simulink model "car_following_model"  (R2017a)
settings: Solver=FixedStepAuto  StartTime=0.0  StopTime=70  FixedStep=.001  RelTol=1e-3
model workspace (MAT data in the model file):
  t_0 = 0
values from neighbouring files (symbols this model uses):
  a = a_list(a_i)    [critical_tau_epsilon.m]    (also in platooning_model_implementation.m = 1.4; run_simulink.m = 1)
  a_max = 1    [critical_tau_epsilon.m]    (also in platooning_model_implementation.m; run_simulink.m)
  a_min = -0.5    [critical_tau_epsilon.m]    (also in platooning_model_implementation.m; run_simulink.m)
  b = 2.0    (= 2)    [critical_tau_epsilon.m]    (also in platooning_model_implementation.m; run_simulink.m)
  delta = 4    [critical_tau_epsilon.m]    (also in platooning_model_implementation.m; run_simulink.m)
  l_avg = 4.8    [critical_tau_epsilon.m]    (also in platooning_model_implementation.m; run_simulink.m)
  N = 1000    [critical_tau_epsilon.m]    (also in platooning_model_implementation.m; run_simulink.m)
  s_0 = 2.0    (= 2)    [critical_tau_epsilon.m]    (also in platooning_model_implementation.m; run_simulink.m)
  T = 1.5    [critical_tau_epsilon.m]    (also in platooning_model_implementation.m; run_simulink.m)
  v_0 = 120    [critical_tau_epsilon.m]    (also in platooning_model_implementation.m; run_simulink.m)
undefined symbols (not defined in the file or in its folder): canChannel
libraries: canlib x9, canmsglib x7, simulink x1, dspstat3 x1, dspindex x1
settings Model: Creator=s132652  LastModifiedBy=s132652

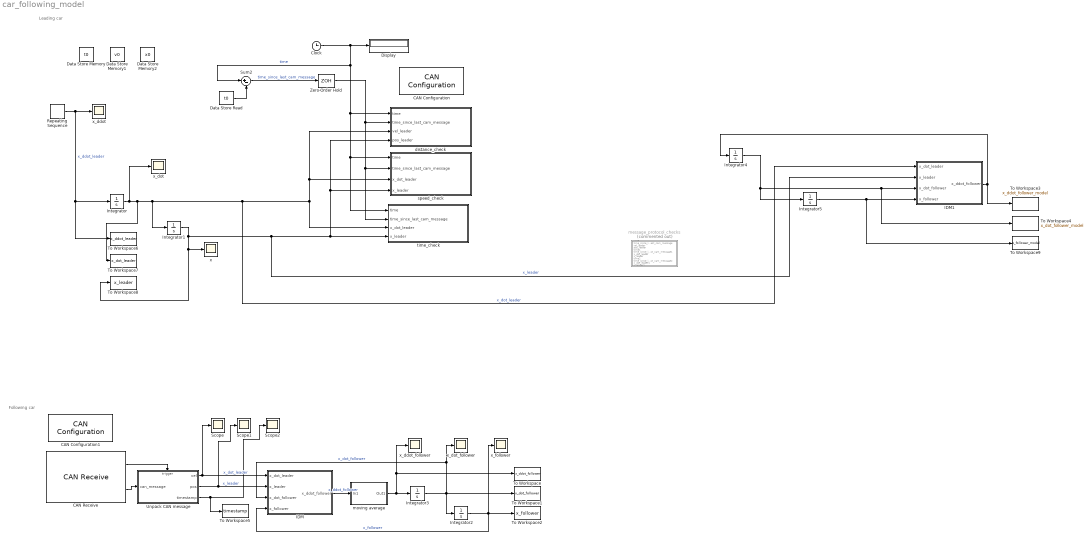
== system car_following_model ==
  note: Leading car
  note: Following car
  CAN Configuration : canlib/CAN Configuration  BlockHandle=5.0001  DeviceMenu=MathWorks Virtual 1 (Channel 1)  Device=MathWorks Virtual 1 (Channel 1)  ObjConstructor=canChannel('MathWorks','Virtual 1',1)  BusSpeed=500000  EnableBitParameters=off  SJW=0  TSEG1=0  TSEG2=0  NSamples=0  AckMode=Normal
      settings: SourceProductName=Vehicle Network Toolbox  SourceProductBaseCode=VN
  CAN Configuration1 : canlib/CAN Configuration  BlockHandle=6.0001  DeviceMenu=MathWorks Virtual 1 (Channel 2)  Device=MathWorks Virtual 1 (Channel 2)  ObjConstructor=canChannel('MathWorks','Virtual 1',2)  BusSpeed=500000  EnableBitParameters=off  SJW=0  TSEG1=0  TSEG2=0  NSamples=0  AckMode=Normal
      settings: SourceProductName=Vehicle Network Toolbox  SourceProductBaseCode=VN
  CAN Receive : canlib/CAN Receive  BlockHandle=7.0001  DeviceMenu=MathWorks Virtual 1 (Channel 2)  Device=MathWorks Virtual 1 (Channel 2)  ObjConstructor=canChannel('MathWorks','Virtual 1',2)  EnableStandardIDsFilter=off  StandardIDs=0  EnableExtendedIDsFilter=off  ExtendedIDs=0  SampleTime=0.01  MsgsPerTimestep=all  StdIDsCombo=Allow all  ExtIDsCombo=Allow all  InternalFilterUpdateStatus=on
      settings: SourceProductName=Vehicle Network Toolbox  SourceProductBaseCode=VN
  Clock : Clock
  Data Store Memory : DataStoreMemory  DataStoreName=t0  ReadBeforeWriteMsg=warning  WriteAfterWriteMsg=warning  WriteAfterReadMsg=warning  ShowAdditionalParam=off
  Data Store Memory1 : DataStoreMemory  DataStoreName=v0  ReadBeforeWriteMsg=warning  WriteAfterWriteMsg=warning  WriteAfterReadMsg=warning  InitialValue=10  ShowAdditionalParam=off
  Data Store Memory2 : DataStoreMemory  DataStoreName=x0  ReadBeforeWriteMsg=warning  WriteAfterWriteMsg=warning  WriteAfterReadMsg=warning  InitialValue=100  ShowAdditionalParam=off
  Data Store Read : DataStoreRead  DataStoreName=t0
  Display : Display
  IDM : Subsystem
  IDM1 : Subsystem
  Integrator : Integrator  InitialCondition=10
  Integrator1 : Integrator  InitialCondition=100
  Integrator2 : Integrator  InitialCondition=76
  Integrator3 : Integrator  InitialCondition=10
  Integrator4 : Integrator  InitialCondition=10
  Integrator5 : Integrator  InitialCondition=78.2
  Repeating Sequence : simulink/Sources/Repeating Sequence  rep_seq_t=[0 5 10 15 20 25 30 35 40 45 50 55 60 65 70]  rep_seq_y=[0 0 0 0 0 a_max a_max 0 0 0 a_min a_min 0 0 0]
  Scope : Scope
  Scope1 : Scope
  Scope2 : Scope
  Sum2 : Sum  Inputs=|+-
  To Workspace : ToWorkspace  VariableName=x_ddot_follower  SaveFormat=Timeseries  SampleTime=-1
  To Workspace1 : ToWorkspace  VariableName=x_dot_follower  SaveFormat=Timeseries  SampleTime=-1
  To Workspace2 : ToWorkspace  VariableName=x_follower  SaveFormat=Timeseries  SampleTime=-1
  To Workspace3 : ToWorkspace  VariableName=x_ddot_follower_model  SaveFormat=Timeseries  SampleTime=-1
  To Workspace4 : ToWorkspace  VariableName=x_dot_follower_model  SaveFormat=Timeseries  SampleTime=-1
  To Workspace5 : ToWorkspace  VariableName=timestamp  SaveFormat=Timeseries  SampleTime=-1
  To Workspace6 : ToWorkspace  VariableName=x_ddot_leader  SaveFormat=Timeseries  SampleTime=-1
  To Workspace7 : ToWorkspace  VariableName=x_dot_leader  SaveFormat=Timeseries  SampleTime=-1
  To Workspace8 : ToWorkspace  VariableName=x_leader  SaveFormat=Timeseries  SampleTime=-1
  To Workspace9 : ToWorkspace  VariableName=x_follower_model  SaveFormat=Timeseries  SampleTime=-1
  Unpack CAN message : Subsystem  TreatAsAtomicUnit=on
  Zero-Order Hold : ZeroOrderHold  SampleTime=0.001
  distance_check : Subsystem
  message_protocol_checks : Subsystem  Commented=on
  moving average : Subsystem
  speed_check : Subsystem
  time_check : Subsystem
  x : Scope
  x_ddot : Scope
  x_ddot_follower : Scope
  x_dot : Scope
  x_dot_follower : Scope
  x_follower : Scope
  wires:
  Repeating Sequence/1 -> To Workspace6/1, Integrator/1, x_ddot/1  "x_ddot_leader"
  Integrator/1 -> x_dot/1, To Workspace7/1, Integrator1/1, IDM1/1(x_dot_leader), distance_check/3(vel_leader), speed_check/3(x_dot_leader), time_check/3(x_dot_leader)  "x_dot_leader"
  Integrator1/1 -> To Workspace8/1, x/1, IDM1/2(x_leader), distance_check/4(pos_leader), speed_check/4(x_leader), time_check/4(x_leader)  "x_leader"
  Clock/1 -> time_check/1(time), speed_check/1(time), distance_check/1(time), Sum2/1, Display/1  "time"
  Data Store Read/1 -> Sum2/2
  Sum2/1 -> Zero-Order Hold/1  "time_since_last_cam_message"
  Zero-Order Hold/1 -> time_check/2(time_since_last_cam_message), speed_check/2(time_since_last_cam_message), distance_check/2(time_since_last_cam_message)
  CAN Receive/2 -> Unpack CAN message/1(can_message)
  CAN Receive/1 -> Unpack CAN message/Trigger
  Unpack CAN message/1(vel) -> IDM/1(x_dot_leader), Scope/1  "x_dot_leader"
  Unpack CAN message/2(pos) -> IDM/2(x_leader), Scope1/1  "x_leader"
  Unpack CAN message/3(timestamp) -> To Workspace5/1, Scope2/1
  IDM/1(x_ddot_follower) -> moving average/1(In1)  "x_ddot_follower"
  moving average/1(Out1) -> To Workspace/1, x_ddot_follower/1, Integrator3/1
  Integrator3/1 -> IDM/3(x_dot_follower), x_dot_follower/1, To Workspace1/1, Integrator2/1  "x_dot_follower"
  Integrator2/1 -> To Workspace2/1, IDM/4(x_follower), x_follower/1  "x_follower"
  Integrator4/1 -> To Workspace4/1, IDM1/3(x_dot_follower), Integrator5/1
  Integrator5/1 -> To Workspace9/1, IDM1/4(x_follower)
  IDM1/1(x_ddot_follower) -> To Workspace3/1, Integrator4/1

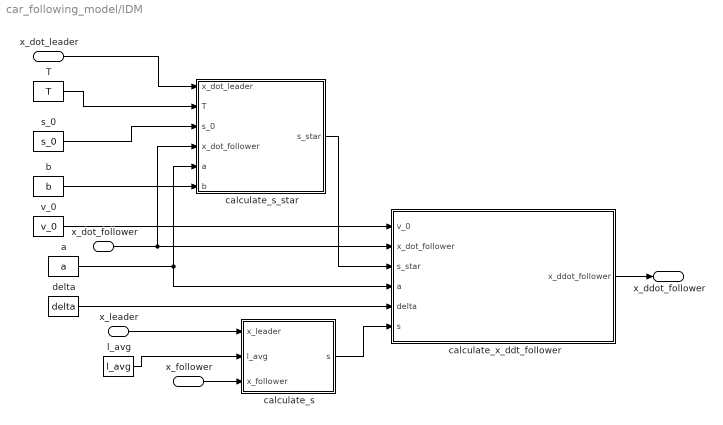
== system car_following_model/IDM ==
  x_dot_leader : Inport
  x_leader : Inport  Port=2
  x_dot_follower : Inport  Port=3
  x_follower : Inport  Port=4
  T : Constant  Value=T
  a : Constant  Value=a
  b : Constant  Value=b
  calculate_s : Subsystem
  calculate_s_star : Subsystem
  calculate_x_ddt_follower : Subsystem
  delta : Constant  Value=delta
  l_avg : Constant  Value=l_avg
  s_0 : Constant  Value=s_0
  v_0 : Constant  Value=v_0
  x_ddot_follower : Outport
  wires:
  v_0/1 -> calculate_x_ddt_follower/1(v_0)
  T/1 -> calculate_s_star/2(T)
  s_0/1 -> calculate_s_star/3(s_0)
  calculate_x_ddt_follower/1(x_ddot_follower) -> x_ddot_follower/1
  b/1 -> calculate_s_star/6(b)
  l_avg/1 -> calculate_s/2(l_avg)
  calculate_s/1(s) -> calculate_x_ddt_follower/6(s)
  delta/1 -> calculate_x_ddt_follower/5(delta)
  calculate_s_star/1(s_star) -> calculate_x_ddt_follower/3(s_star)
  x_follower/1 -> calculate_s/3(x_follower)
  x_dot_leader/1 -> calculate_s_star/1(x_dot_leader)
  x_leader/1 -> calculate_s/1(x_leader)
  x_dot_follower/1 -> calculate_s_star/4(x_dot_follower), calculate_x_ddt_follower/2(x_dot_follower)
  a/1 -> calculate_x_ddt_follower/4(a), calculate_s_star/5(a)

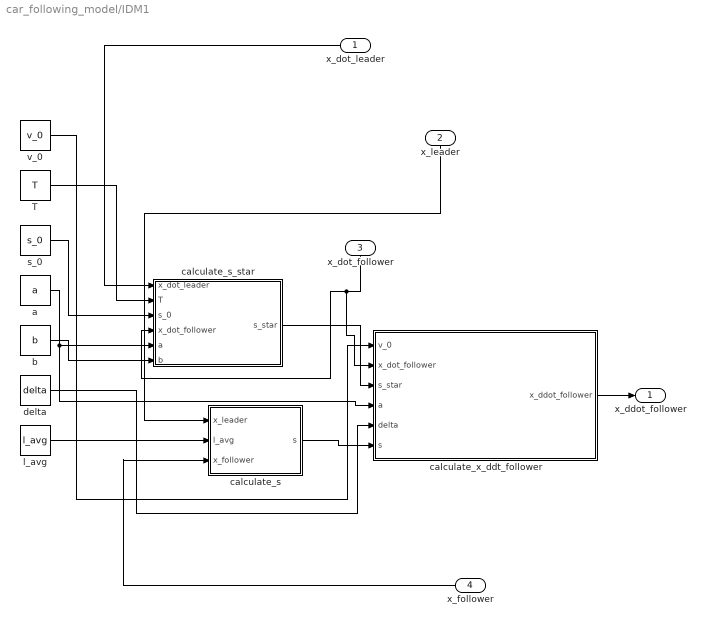
== system car_following_model/IDM1 ==
  x_dot_leader : Inport
  x_leader : Inport  Port=2
  x_dot_follower : Inport  Port=3
  x_follower : Inport  Port=4
  T : Constant  Value=T
  a : Constant  Value=a
  b : Constant  Value=b
  calculate_s : Subsystem
  calculate_s_star : Subsystem
  calculate_x_ddt_follower : Subsystem
  delta : Constant  Value=delta
  l_avg : Constant  Value=l_avg
  "s_0 " : Constant  Value=s_0
  v_0 : Constant  Value=v_0
  x_ddot_follower : Outport
  wires:
  a/1 -> calculate_x_ddt_follower/4(a), calculate_s_star/5(a)
  v_0/1 -> calculate_x_ddt_follower/1(v_0)
  T/1 -> calculate_s_star/2(T)
  "s_0 "/1 -> calculate_s_star/3(s_0)
  calculate_x_ddt_follower/1(x_ddot_follower) -> x_ddot_follower/1
  b/1 -> calculate_s_star/6(b)
  l_avg/1 -> calculate_s/2(l_avg)
  calculate_s/1(s) -> calculate_x_ddt_follower/6(s)
  delta/1 -> calculate_x_ddt_follower/5(delta)
  calculate_s_star/1(s_star) -> calculate_x_ddt_follower/3(s_star)
  x_follower/1 -> calculate_s/3(x_follower)
  x_dot_follower/1 -> calculate_x_ddt_follower/2(x_dot_follower), calculate_s_star/4(x_dot_follower)
  x_dot_leader/1 -> calculate_s_star/1(x_dot_leader)
  x_leader/1 -> calculate_s/1(x_leader)

== system car_following_model/Unpack CAN message ==
  can_message : Inport
  function : TriggerPort  TriggerType=function-call  VariantControl=Variant
  CAN Unpack : canmsglib/CAN Unpack  MsgList=(none)  MsgName=CAN Msg  MsgIDType=Standard (11-bit identifier)  MsgIdentifier=0  MsgLength=8  SignalInfo=position_leader$0$16$1$1$1$0$0.1$0$-Inf$Inf$#velocity_leader$16$16$1$1$1$0$0.0025$0$-Inf$Inf$#timestamp$32$16$1$1$1$0$0.01$0$-Inf$Inf$#  NSignals=3  IDPort=off  TimestampPort=off  ErrorPort=off  RemotePort=off  LengthPort=off  StatusPort=off  StartBits=str2num('[int32(0);int32(16);int32(32)]')  SignalSizes=str2num('[int32(16);int32(16);int32(16)]')  ByteOrders=str2num('[int32(1);int32(1);int32(1)]')  DataTypes=str2num('[int32(1);int32(1);int32(1)]')  MultiplexTypes=str2num('[int32(1);int32(1);int32(1)]')  MultiplexValues=str2num('[double(0);double(0);double(0)]')  Factors=str2num('[double(0.1);double(0.0025);double(0.01)]')  Offsets=str2num('[double(0);double(0);double(0)]')  Minimums=str2num('[double(-Inf);double(-Inf);double(-Inf)]')  Maximums=str2num('[double(Inf);double(Inf);double(Inf)]')  ApplyMinMax=off
      settings: SourceProductName=Simulink Real-Time
  vel : Outport
  pos : Outport  Port=2
  timestamp : Outport  Port=3
  wires:
  can_message/1 -> CAN Unpack/1
  CAN Unpack/2 -> vel/1
  CAN Unpack/1 -> pos/1
  CAN Unpack/3 -> timestamp/1

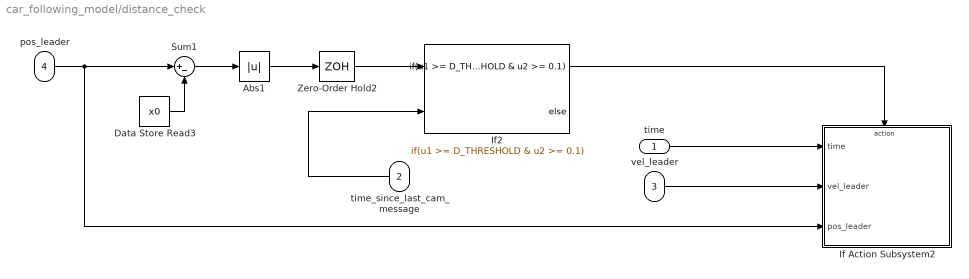
== system car_following_model/distance_check ==
  time : Inport
  time_since_last_cam_message : Inport  Port=2
  vel_leader : Inport  Port=3
  pos_leader : Inport  Port=4
  Abs1 : Abs
  Data Store Read3 : DataStoreRead  DataStoreName=x0
  If Action Subsystem2 : Subsystem  TreatAsAtomicUnit=on
  If2 : If  NumInputs=2  IfExpression=u1 >= D_THRESHOLD & u2 >= 0.1
  Sum1 : Sum  Inputs=|+-
  Zero-Order Hold2 : ZeroOrderHold  SampleTime=0.001
  wires:
  Data Store Read3/1 -> Sum1/2
  Sum1/1 -> Abs1/1
  Abs1/1 -> Zero-Order Hold2/1
  Zero-Order Hold2/1 -> If2/1
  If2/1 -> If Action Subsystem2/Action
  time_since_last_cam_message/1 -> If2/2
  time/1 -> If Action Subsystem2/1(time)
  pos_leader/1 -> If Action Subsystem2/3(pos_leader), Sum1/1
  vel_leader/1 -> If Action Subsystem2/2(vel_leader)

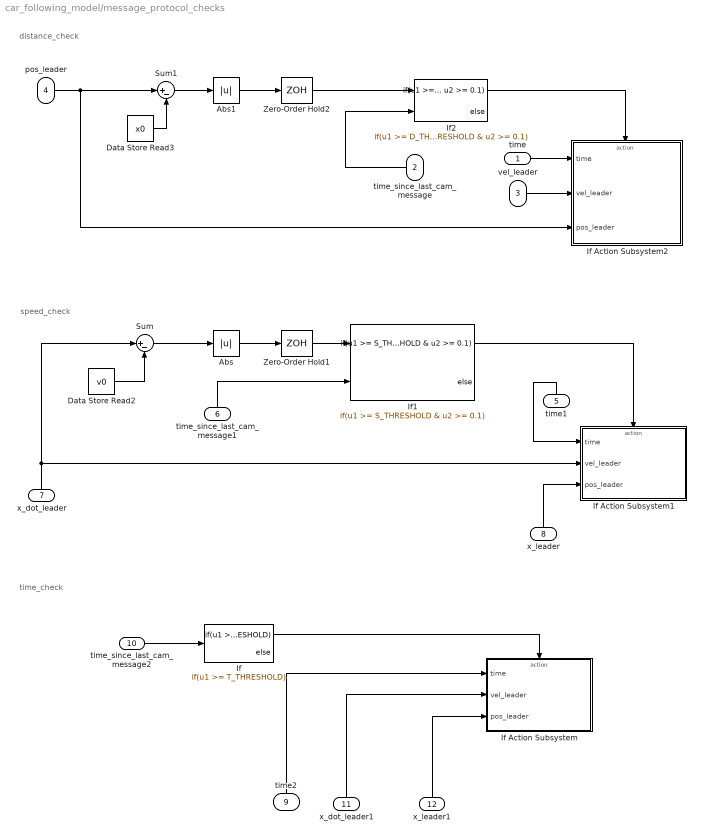
== system car_following_model/message_protocol_checks ==
  note: time_check
  note: speed_check
  note: distance_check
  time : Inport
  time_since_last_cam_message : Inport  Port=2
  vel_leader : Inport  Port=3
  pos_leader : Inport  Port=4
  time1 : Inport  Port=5
  time_since_last_cam_message1 : Inport  Port=6
  x_dot_leader : Inport  Port=7
  x_leader : Inport  Port=8
  time2 : Inport  Port=9
  time_since_last_cam_message2 : Inport  Port=10
  x_dot_leader1 : Inport  Port=11
  x_leader1 : Inport  Port=12
  Abs : Abs
  Abs1 : Abs
  Data Store Read2 : DataStoreRead  DataStoreName=v0
  Data Store Read3 : DataStoreRead  DataStoreName=x0
  If : If  IfExpression=u1 >= T_THRESHOLD
  If Action Subsystem : Subsystem  TreatAsAtomicUnit=on
  If Action Subsystem1 : Subsystem  TreatAsAtomicUnit=on
  If Action Subsystem2 : Subsystem  TreatAsAtomicUnit=on
  If1 : If  NumInputs=2  IfExpression=u1 >= S_THRESHOLD & u2 >= 0.1
  If2 : If  NumInputs=2  IfExpression=u1 >= D_THRESHOLD & u2 >= 0.1
  Sum : Sum  Inputs=|+-
  Sum1 : Sum  Inputs=|+-
  Zero-Order Hold1 : ZeroOrderHold  SampleTime=0.001
  Zero-Order Hold2 : ZeroOrderHold  SampleTime=0.001
  wires:
  time_since_last_cam_message/1 -> If2/2
  If2/1 -> If Action Subsystem2/Action
  Sum1/1 -> Abs1/1
  time/1 -> If Action Subsystem2/1(time)
  Zero-Order Hold2/1 -> If2/1
  Abs1/1 -> Zero-Order Hold2/1
  pos_leader/1 -> If Action Subsystem2/3(pos_leader), Sum1/1
  Data Store Read3/1 -> Sum1/2
  vel_leader/1 -> If Action Subsystem2/2(vel_leader)
  Abs/1 -> Zero-Order Hold1/1
  time1/1 -> If Action Subsystem1/1(time)
  x_dot_leader/1 -> Sum/1, If Action Subsystem1/2(vel_leader)
  Zero-Order Hold1/1 -> If1/1
  Sum/1 -> Abs/1
  Data Store Read2/1 -> Sum/2
  x_leader/1 -> If Action Subsystem1/3(pos_leader)
  time_since_last_cam_message1/1 -> If1/2
  If1/1 -> If Action Subsystem1/Action
  time2/1 -> If Action Subsystem/1(time)
  x_dot_leader1/1 -> If Action Subsystem/2(vel_leader)
  If/1 -> If Action Subsystem/Action
  x_leader1/1 -> If Action Subsystem/3(pos_leader)
  time_since_last_cam_message2/1 -> If/1

== system car_following_model/moving average ==
  note: moving average
  In1 : Inport
  IC : InitialCondition  Value=zeros(N,1)
  Mean : dspstat3/Mean  run=off  reset_popup=None  InputProcessing=Columns as channels (frame based)  directionMode=Each column  dimension=1  roiEnable=off  roiType=Rectangles  roiPortion=Entire ROI  roiOutput=Individual statistics for each ROI  roiFlag=off  outputDataTypeStr=Inherit: Same as accumulator  outputLastDataTypeStr=Inherit: Same as accumulator  outputMin=[]  outputMax=[]  roundingMode=Floor  overflowMode=off
  Memory : Memory
  Mux : Mux  Inputs=2
  Variable Selector : dspindex/Variable Selector  NumInputs=1  rowsOrCols=Rows  IdxMode=Fixed  Elements=1:N-1  ZerOneIdxMode=One-based  errmode=Clip Index  FillMode=on  FillValues=0
  Out1 : Outport
  wires:
  In1/1 -> Mux/1
  Mux/1 -> Mean/1, Memory/1
  Memory/1 -> IC/1
  IC/1 -> Variable Selector/1
  Mean/1 -> Out1/1
  Variable Selector/1 -> Mux/2

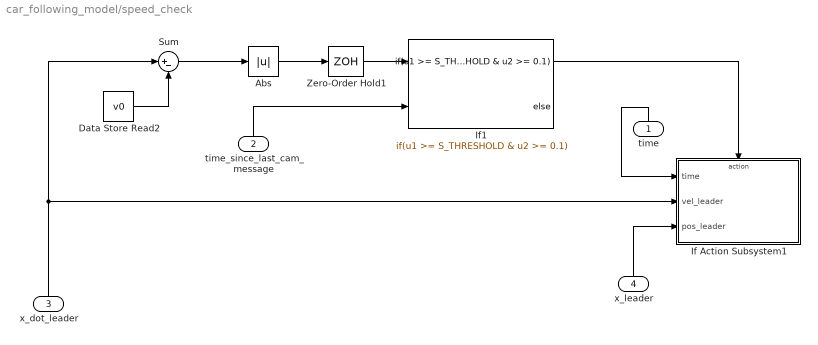
== system car_following_model/speed_check ==
  time : Inport
  time_since_last_cam_message : Inport  Port=2
  x_dot_leader : Inport  Port=3
  x_leader : Inport  Port=4
  Abs : Abs
  Data Store Read2 : DataStoreRead  DataStoreName=v0
  If Action Subsystem1 : Subsystem  TreatAsAtomicUnit=on
  If1 : If  NumInputs=2  IfExpression=u1 >= S_THRESHOLD & u2 >= 0.1
  Sum : Sum  Inputs=|+-
  Zero-Order Hold1 : ZeroOrderHold  SampleTime=0.001
  wires:
  Data Store Read2/1 -> Sum/2
  Sum/1 -> Abs/1
  Abs/1 -> Zero-Order Hold1/1
  If1/1 -> If Action Subsystem1/Action
  Zero-Order Hold1/1 -> If1/1
  time/1 -> If Action Subsystem1/1(time)
  x_dot_leader/1 -> Sum/1, If Action Subsystem1/2(vel_leader)
  x_leader/1 -> If Action Subsystem1/3(pos_leader)
  time_since_last_cam_message/1 -> If1/2

== system car_following_model/time_check ==
  time : Inport
  time_since_last_cam_message : Inport  Port=2
  x_dot_leader : Inport  Port=3
  x_leader : Inport  Port=4
  If : If  IfExpression=u1 >= T_THRESHOLD
  If Action Subsystem : Subsystem  TreatAsAtomicUnit=on
  wires:
  If/1 -> If Action Subsystem/Action
  time_since_last_cam_message/1 -> If/1
  time/1 -> If Action Subsystem/1(time)
  x_dot_leader/1 -> If Action Subsystem/2(vel_leader)
  x_leader/1 -> If Action Subsystem/3(pos_leader)

== system car_following_model/IDM/calculate_s ==
  x_leader : Inport
  l_avg : Inport  Port=2
  x_follower : Inport  Port=3
  Sum3 : Sum  Inputs=|+-
  Sum4 : Sum  Inputs=|+-
  s : Outport
  wires:
  Sum4/1 -> s/1  "s"
  Sum3/1 -> Sum4/1
  l_avg/1 -> Sum4/2
  x_follower/1 -> Sum3/2
  x_leader/1 -> Sum3/1

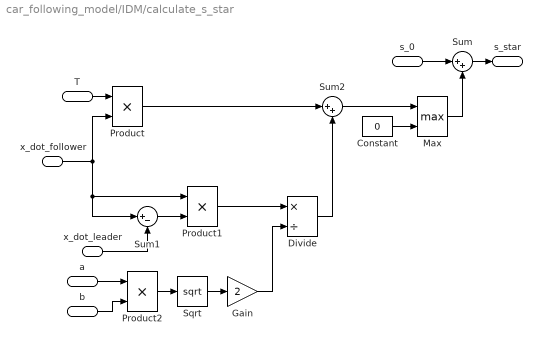
== system car_following_model/IDM/calculate_s_star ==
  x_dot_leader : Inport
  T : Inport  Port=2
  s_0 : Inport  Port=3
  x_dot_follower : Inport  Port=4
  a : Inport  Port=5
  b : Inport  Port=6
  Constant : Constant  Value=0
  Divide : Product  Inputs=*/
  Gain : Gain  Gain=2
  Max : MinMax  Function=max  Inputs=2
  Product : Product
  Product1 : Product
  Product2 : Product
  Sqrt : Sqrt  SaturateOnIntegerOverflow=on
  Sum : Sum  Inputs=|++
  Sum1 : Sum  Inputs=|+-
  Sum2 : Sum  Inputs=|++
  s_star : Outport
  wires:
  Sum1/1 -> Product1/2
  T/1 -> Product/1
  s_0/1 -> Sum/1
  Product1/1 -> Divide/1
  Product/1 -> Sum2/1
  Divide/1 -> Sum2/2
  x_dot_leader/1 -> Sum1/2
  Product2/1 -> Sqrt/1
  Sqrt/1 -> Gain/1
  Gain/1 -> Divide/2
  a/1 -> Product2/1
  b/1 -> Product2/2
  Constant/1 -> Max/2
  Sum2/1 -> Max/1
  Max/1 -> Sum/2
  Sum/1 -> s_star/1
  x_dot_follower/1 -> Product/2, Product1/1, Sum1/1

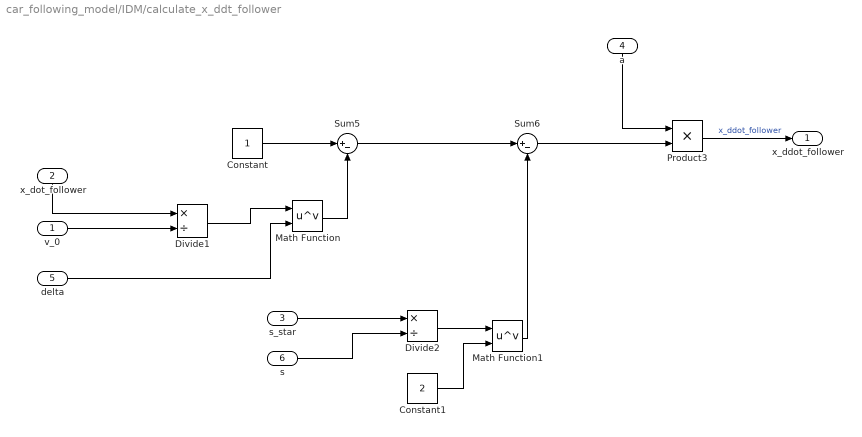
== system car_following_model/IDM/calculate_x_ddt_follower ==
  v_0 : Inport
  x_dot_follower : Inport  Port=2
  s_star : Inport  Port=3
  a : Inport  Port=4
  delta : Inport  Port=5
  s : Inport  Port=6
  Constant : Constant
  Constant1 : Constant  Value=2
  Divide1 : Product  Inputs=*/
  Divide2 : Product  Inputs=*/
  Math Function : Math  Operator=pow  SaturateOnIntegerOverflow=on
  Math Function1 : Math  Operator=pow  SaturateOnIntegerOverflow=on
  Product3 : Product
  Sum5 : Sum  Inputs=|+-
  Sum6 : Sum  Inputs=|+-
  x_ddot_follower : Outport
  wires:
  Product3/1 -> x_ddot_follower/1  "x_ddot_follower"
  v_0/1 -> Divide1/2
  Constant/1 -> Sum5/1
  Math Function/1 -> Sum5/2
  a/1 -> Product3/1
  x_dot_follower/1 -> Divide1/1
  s/1 -> Divide2/2
  s_star/1 -> Divide2/1
  Sum5/1 -> Sum6/1
  Constant1/1 -> Math Function1/2
  Divide1/1 -> Math Function/1
  Math Function1/1 -> Sum6/2
  delta/1 -> Math Function/2
  Divide2/1 -> Math Function1/1
  Sum6/1 -> Product3/2

== system car_following_model/IDM1/calculate_s ==
  x_leader : Inport
  l_avg : Inport  Port=2
  x_follower : Inport  Port=3
  Sum3 : Sum  Inputs=|+-
  Sum4 : Sum  Inputs=|+-
  s : Outport
  wires:
  Sum4/1 -> s/1  "s"
  Sum3/1 -> Sum4/1
  l_avg/1 -> Sum4/2
  x_follower/1 -> Sum3/2
  x_leader/1 -> Sum3/1

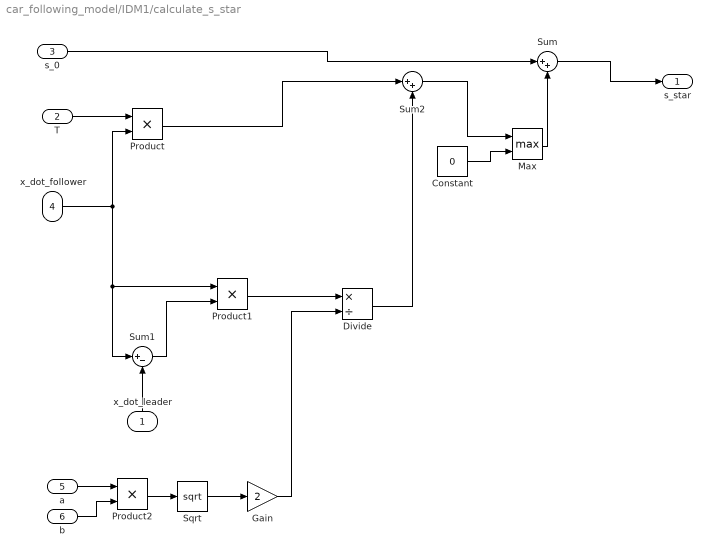
== system car_following_model/IDM1/calculate_s_star ==
  x_dot_leader : Inport
  T : Inport  Port=2
  s_0 : Inport  Port=3
  x_dot_follower : Inport  Port=4
  a : Inport  Port=5
  b : Inport  Port=6
  Constant : Constant  Value=0
  Divide : Product  Inputs=*/
  Gain : Gain  Gain=2
  Max : MinMax  Function=max  Inputs=2
  Product : Product
  Product1 : Product
  Product2 : Product
  Sqrt : Sqrt  SaturateOnIntegerOverflow=on
  Sum : Sum  Inputs=|++
  Sum1 : Sum  Inputs=|+-
  Sum2 : Sum  Inputs=|++
  s_star : Outport
  wires:
  Sum1/1 -> Product1/2
  T/1 -> Product/1
  s_0/1 -> Sum/1
  Product1/1 -> Divide/1
  Product/1 -> Sum2/1
  Divide/1 -> Sum2/2
  x_dot_leader/1 -> Sum1/2
  x_dot_follower/1 -> Product/2, Sum1/1, Product1/1
  Product2/1 -> Sqrt/1
  Sqrt/1 -> Gain/1
  Gain/1 -> Divide/2
  a/1 -> Product2/1
  b/1 -> Product2/2
  Constant/1 -> Max/2
  Sum2/1 -> Max/1
  Max/1 -> Sum/2
  Sum/1 -> s_star/1

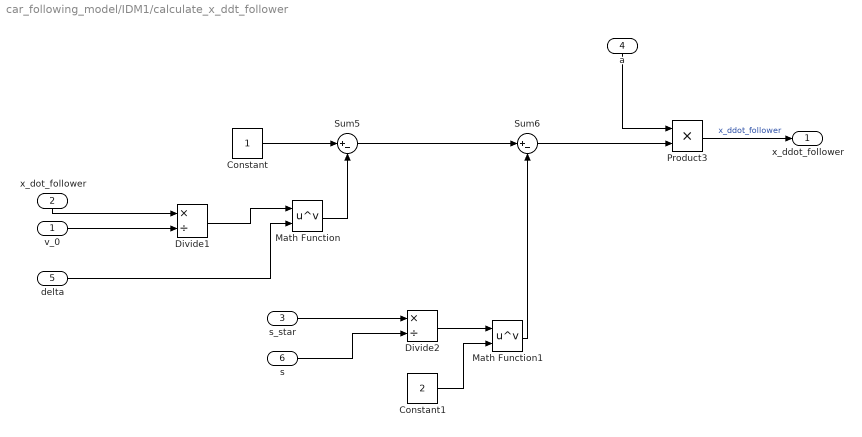
== system car_following_model/IDM1/calculate_x_ddt_follower ==
  v_0 : Inport
  x_dot_follower : Inport  Port=2
  s_star : Inport  Port=3
  a : Inport  Port=4
  delta : Inport  Port=5
  s : Inport  Port=6
  Constant : Constant
  Constant1 : Constant  Value=2
  Divide1 : Product  Inputs=*/
  Divide2 : Product  Inputs=*/
  Math Function : Math  Operator=pow  SaturateOnIntegerOverflow=on
  Math Function1 : Math  Operator=pow  SaturateOnIntegerOverflow=on
  Product3 : Product
  Sum5 : Sum  Inputs=|+-
  Sum6 : Sum  Inputs=|+-
  x_ddot_follower : Outport
  wires:
  Product3/1 -> x_ddot_follower/1  "x_ddot_follower"
  v_0/1 -> Divide1/2
  Constant/1 -> Sum5/1
  Math Function/1 -> Sum5/2
  a/1 -> Product3/1
  x_dot_follower/1 -> Divide1/1
  s/1 -> Divide2/2
  s_star/1 -> Divide2/1
  Sum5/1 -> Sum6/1
  Constant1/1 -> Math Function1/2
  Divide1/1 -> Math Function/1
  Math Function1/1 -> Sum6/2
  delta/1 -> Math Function/2
  Divide2/1 -> Math Function1/1
  Sum6/1 -> Product3/2

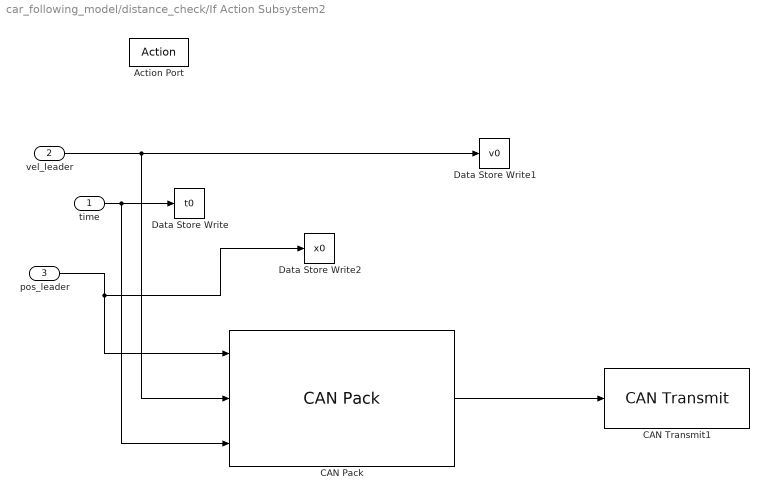
== system car_following_model/distance_check/If Action Subsystem2 ==
  time : Inport
  vel_leader : Inport  Port=2
  pos_leader : Inport  Port=3
  Action Port : ActionPort  ActionType=then
  CAN Pack : canmsglib/CAN Pack  MsgList=(none)  MsgName=CAN Msg  MsgIDType=Standard (11-bit identifier)  MsgIdentifier=0  MsgLength=8  SignalInfo=position_leader$0$16$1$1$1$0$0.1$0$-Inf$Inf$#velocity_leader$16$16$1$1$1$0$0.0025$0$-Inf$Inf$#timestamp$32$16$1$1$1$0$0.01$0$-Inf$Inf$#  NSignals=3  StartBits=str2num('[int32(0);int32(16);int32(32)]')  SignalSizes=str2num('[int32(16);int32(16);int32(16)]')  ByteOrders=str2num('[int32(1);int32(1);int32(1)]')  DataTypes=str2num('[int32(1);int32(1);int32(1)]')  MultiplexTypes=str2num('[int32(1);int32(1);int32(1)]')  MultiplexValues=str2num('[double(0);double(0);double(0)]')  Factors=str2num('[double(0.1);double(0.0025);double(0.01)]')  Offsets=str2num('[double(0);double(0);double(0)]')  Minimums=str2num('[double(-Inf);double(-Inf);double(-Inf)]')  Maximums=str2num('[double(Inf);double(Inf);double(Inf)]')  Remote=off  ApplyMinMax=off
      settings: SourceProductName=Simulink Real-Time  DataFormat=manually specified signals
  CAN Transmit1 : canlib/CAN Transmit  BlockHandle=170.0001  DeviceMenu=MathWorks Virtual 1 (Channel 1)  Device=MathWorks Virtual 1 (Channel 1)  ObjConstructor=canChannel('MathWorks','Virtual 1',1)  EnablePeriodicTransmit=off  MessagePeriod=1.000
      settings: SourceProductName=Vehicle Network Toolbox  SourceProductBaseCode=VN
  Data Store Write : DataStoreWrite  DataStoreName=t0
  Data Store Write1 : DataStoreWrite  DataStoreName=v0
  Data Store Write2 : DataStoreWrite  DataStoreName=x0
  wires:
  time/1 -> CAN Pack/3, Data Store Write/1
  vel_leader/1 -> CAN Pack/2, Data Store Write1/1
  CAN Pack/1 -> CAN Transmit1/1
  pos_leader/1 -> Data Store Write2/1, CAN Pack/1

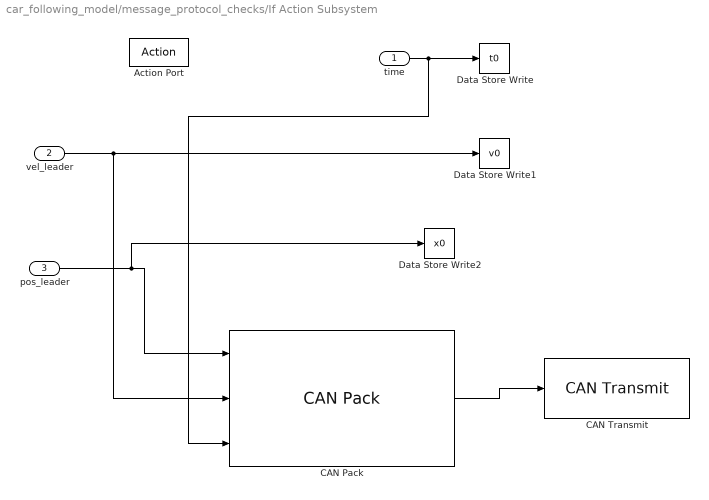
== system car_following_model/message_protocol_checks/If Action Subsystem ==
  time : Inport
  vel_leader : Inport  Port=2
  pos_leader : Inport  Port=3
  Action Port : ActionPort  ActionType=then
  CAN Pack : canmsglib/CAN Pack  MsgList=(none)  MsgName=CAN Msg  MsgIDType=Standard (11-bit identifier)  MsgIdentifier=0  MsgLength=8  SignalInfo=position_leader$0$16$1$1$1$0$0.1$3212$-Inf$Inf$#velocity_leader$16$16$1$1$1$0$0.0025$0$-Inf$Inf$#timestamp$32$16$1$1$1$0$0.01$0$-Inf$Inf$#  NSignals=3  StartBits=str2num('[int32(0);int32(16);int32(32)]')  SignalSizes=str2num('[int32(16);int32(16);int32(16)]')  ByteOrders=str2num('[int32(1);int32(1);int32(1)]')  DataTypes=str2num('[int32(1);int32(1);int32(1)]')  MultiplexTypes=str2num('[int32(1);int32(1);int32(1)]')  MultiplexValues=str2num('[double(0);double(0);double(0)]')  Factors=str2num('[double(0.1);double(0.0025);double(0.01)]')  Offsets=str2num('[double(3212);double(0);double(0)]')  Minimums=str2num('[double(-Inf);double(-Inf);double(-Inf)]')  Maximums=str2num('[double(Inf);double(Inf);double(Inf)]')  Remote=off  ApplyMinMax=off
      settings: SourceProductName=Simulink Real-Time  DataFormat=manually specified signals
  CAN Transmit : canlib/CAN Transmit  BlockHandle=271.0001  DeviceMenu=MathWorks Virtual 1 (Channel 1)  Device=MathWorks Virtual 1 (Channel 1)  ObjConstructor=canChannel('MathWorks','Virtual 1',1)  EnablePeriodicTransmit=off  MessagePeriod=1.000
      settings: SourceProductName=Vehicle Network Toolbox  SourceProductBaseCode=VN
  Data Store Write : DataStoreWrite  DataStoreName=t0
  Data Store Write1 : DataStoreWrite  DataStoreName=v0
  Data Store Write2 : DataStoreWrite  DataStoreName=x0
  wires:
  time/1 -> CAN Pack/3, Data Store Write/1
  vel_leader/1 -> CAN Pack/2, Data Store Write1/1
  CAN Pack/1 -> CAN Transmit/1
  pos_leader/1 -> Data Store Write2/1, CAN Pack/1

== system car_following_model/message_protocol_checks/If Action Subsystem1 ==
  time : Inport
  vel_leader : Inport  Port=2
  pos_leader : Inport  Port=3
  Action Port : ActionPort  ActionType=then
  CAN Pack : canmsglib/CAN Pack  MsgList=(none)  MsgName=CAN Msg  MsgIDType=Standard (11-bit identifier)  MsgIdentifier=0  MsgLength=8  SignalInfo=position_leader$0$16$1$1$1$0$0.1$3212$-Inf$Inf$#velocity_leader$16$16$1$1$1$0$0.0025$0$-Inf$Inf$#timestamp$32$16$1$1$1$0$0.01$0$-Inf$Inf$#  NSignals=3  StartBits=str2num('[int32(0);int32(16);int32(32)]')  SignalSizes=str2num('[int32(16);int32(16);int32(16)]')  ByteOrders=str2num('[int32(1);int32(1);int32(1)]')  DataTypes=str2num('[int32(1);int32(1);int32(1)]')  MultiplexTypes=str2num('[int32(1);int32(1);int32(1)]')  MultiplexValues=str2num('[double(0);double(0);double(0)]')  Factors=str2num('[double(0.1);double(0.0025);double(0.01)]')  Offsets=str2num('[double(3212);double(0);double(0)]')  Minimums=str2num('[double(-Inf);double(-Inf);double(-Inf)]')  Maximums=str2num('[double(Inf);double(Inf);double(Inf)]')  Remote=off  ApplyMinMax=off
      settings: SourceProductName=Simulink Real-Time  DataFormat=manually specified signals
  CAN Transmit : canlib/CAN Transmit  BlockHandle=231.0001  DeviceMenu=MathWorks Virtual 1 (Channel 1)  Device=MathWorks Virtual 1 (Channel 1)  ObjConstructor=canChannel('MathWorks','Virtual 1',1)  EnablePeriodicTransmit=off  MessagePeriod=1.000
      settings: SourceProductName=Vehicle Network Toolbox  SourceProductBaseCode=VN
  Data Store Write : DataStoreWrite  DataStoreName=t0
  Data Store Write1 : DataStoreWrite  DataStoreName=v0
  Data Store Write2 : DataStoreWrite  DataStoreName=x0
  wires:
  time/1 -> CAN Pack/3, Data Store Write/1
  vel_leader/1 -> CAN Pack/2, Data Store Write1/1
  CAN Pack/1 -> CAN Transmit/1
  pos_leader/1 -> Data Store Write2/1, CAN Pack/1

== system car_following_model/message_protocol_checks/If Action Subsystem2 ==
  time : Inport
  vel_leader : Inport  Port=2
  pos_leader : Inport  Port=3
  Action Port : ActionPort  ActionType=then
  CAN Pack : canmsglib/CAN Pack  MsgList=(none)  MsgName=CAN Msg  MsgIDType=Standard (11-bit identifier)  MsgIdentifier=0  MsgLength=8  SignalInfo=position_leader$0$16$1$1$1$0$0.1$3212$-Inf$Inf$#velocity_leader$16$16$1$1$1$0$0.0025$0$-Inf$Inf$#timestamp$32$16$1$1$1$0$0.01$0$-Inf$Inf$#  NSignals=3  StartBits=str2num('[int32(0);int32(16);int32(32)]')  SignalSizes=str2num('[int32(16);int32(16);int32(16)]')  ByteOrders=str2num('[int32(1);int32(1);int32(1)]')  DataTypes=str2num('[int32(1);int32(1);int32(1)]')  MultiplexTypes=str2num('[int32(1);int32(1);int32(1)]')  MultiplexValues=str2num('[double(0);double(0);double(0)]')  Factors=str2num('[double(0.1);double(0.0025);double(0.01)]')  Offsets=str2num('[double(3212);double(0);double(0)]')  Minimums=str2num('[double(-Inf);double(-Inf);double(-Inf)]')  Maximums=str2num('[double(Inf);double(Inf);double(Inf)]')  Remote=off  ApplyMinMax=off
      settings: SourceProductName=Simulink Real-Time  DataFormat=manually specified signals
  CAN Transmit1 : canlib/CAN Transmit  BlockHandle=174.0001  DeviceMenu=MathWorks Virtual 1 (Channel 1)  Device=MathWorks Virtual 1 (Channel 1)  ObjConstructor=canChannel('MathWorks','Virtual 1',1)  EnablePeriodicTransmit=off  MessagePeriod=1.000
      settings: SourceProductName=Vehicle Network Toolbox  SourceProductBaseCode=VN
  Data Store Write : DataStoreWrite  DataStoreName=t0
  Data Store Write1 : DataStoreWrite  DataStoreName=v0
  Data Store Write2 : DataStoreWrite  DataStoreName=x0
  wires:
  time/1 -> CAN Pack/3, Data Store Write/1
  vel_leader/1 -> CAN Pack/2, Data Store Write1/1
  CAN Pack/1 -> CAN Transmit1/1
  pos_leader/1 -> Data Store Write2/1, CAN Pack/1

== system car_following_model/speed_check/If Action Subsystem1 ==
  time : Inport
  vel_leader : Inport  Port=2
  pos_leader : Inport  Port=3
  Action Port : ActionPort  ActionType=then
  CAN Pack : canmsglib/CAN Pack  MsgList=(none)  MsgName=CAN Msg  MsgIDType=Standard (11-bit identifier)  MsgIdentifier=0  MsgLength=8  SignalInfo=position_leader$0$16$1$1$1$0$0.1$0$-Inf$Inf$#velocity_leader$16$16$1$1$1$0$0.0025$0$-Inf$Inf$#timestamp$32$16$1$1$1$0$0.01$0$-Inf$Inf$#  NSignals=3  StartBits=str2num('[int32(0);int32(16);int32(32)]')  SignalSizes=str2num('[int32(16);int32(16);int32(16)]')  ByteOrders=str2num('[int32(1);int32(1);int32(1)]')  DataTypes=str2num('[int32(1);int32(1);int32(1)]')  MultiplexTypes=str2num('[int32(1);int32(1);int32(1)]')  MultiplexValues=str2num('[double(0);double(0);double(0)]')  Factors=str2num('[double(0.1);double(0.0025);double(0.01)]')  Offsets=str2num('[double(0);double(0);double(0)]')  Minimums=str2num('[double(-Inf);double(-Inf);double(-Inf)]')  Maximums=str2num('[double(Inf);double(Inf);double(Inf)]')  Remote=off  ApplyMinMax=off
      settings: SourceProductName=Simulink Real-Time  DataFormat=manually specified signals
  CAN Transmit : canlib/CAN Transmit  BlockHandle=342.0001  DeviceMenu=MathWorks Virtual 1 (Channel 1)  Device=MathWorks Virtual 1 (Channel 1)  ObjConstructor=canChannel('MathWorks','Virtual 1',1)  EnablePeriodicTransmit=off  MessagePeriod=1.000
      settings: SourceProductName=Vehicle Network Toolbox  SourceProductBaseCode=VN
  Data Store Write : DataStoreWrite  DataStoreName=t0
  Data Store Write1 : DataStoreWrite  DataStoreName=v0
  Data Store Write2 : DataStoreWrite  DataStoreName=x0
  wires:
  time/1 -> CAN Pack/3, Data Store Write/1
  vel_leader/1 -> CAN Pack/2, Data Store Write1/1
  CAN Pack/1 -> CAN Transmit/1
  pos_leader/1 -> Data Store Write2/1, CAN Pack/1

== system car_following_model/time_check/If Action Subsystem ==
  time : Inport
  vel_leader : Inport  Port=2
  pos_leader : Inport  Port=3
  Action Port : ActionPort  ActionType=then
  CAN Pack : canmsglib/CAN Pack  MsgList=(none)  MsgName=CAN Msg  MsgIDType=Standard (11-bit identifier)  MsgIdentifier=0  MsgLength=8  SignalInfo=position_leader$0$16$1$1$1$0$0.1$0$-Inf$Inf$#velocity_leader$16$16$1$1$1$0$0.0025$0$-Inf$Inf$#timestamp$32$16$1$1$1$0$0.01$0$-Inf$Inf$#  NSignals=3  StartBits=str2num('[int32(0);int32(16);int32(32)]')  SignalSizes=str2num('[int32(16);int32(16);int32(16)]')  ByteOrders=str2num('[int32(1);int32(1);int32(1)]')  DataTypes=str2num('[int32(1);int32(1);int32(1)]')  MultiplexTypes=str2num('[int32(1);int32(1);int32(1)]')  MultiplexValues=str2num('[double(0);double(0);double(0)]')  Factors=str2num('[double(0.1);double(0.0025);double(0.01)]')  Offsets=str2num('[double(0);double(0);double(0)]')  Minimums=str2num('[double(-Inf);double(-Inf);double(-Inf)]')  Maximums=str2num('[double(Inf);double(Inf);double(Inf)]')  Remote=off  ApplyMinMax=off
      settings: SourceProductName=Simulink Real-Time  DataFormat=manually specified signals
  CAN Transmit : canlib/CAN Transmit  BlockHandle=382.0001  DeviceMenu=MathWorks Virtual 1 (Channel 1)  Device=MathWorks Virtual 1 (Channel 1)  ObjConstructor=canChannel('MathWorks','Virtual 1',1)  EnablePeriodicTransmit=off  MessagePeriod=1.000
      settings: SourceProductName=Vehicle Network Toolbox  SourceProductBaseCode=VN
  Data Store Write : DataStoreWrite  DataStoreName=t0
  Data Store Write1 : DataStoreWrite  DataStoreName=v0
  Data Store Write2 : DataStoreWrite  DataStoreName=x0
  wires:
  time/1 -> CAN Pack/3, Data Store Write/1
  vel_leader/1 -> CAN Pack/2, Data Store Write1/1
  CAN Pack/1 -> CAN Transmit/1
  pos_leader/1 -> Data Store Write2/1, CAN Pack/1
